simulink model "RVC_Joint_space_PD_control_gravity_compensation"  (R2020b)
settings: Solver=VariableStepAuto  StartTime=0.0  StopTime=10  RelTol=1e-3
values from neighbouring files (symbols this model uses):
  dotqd = [0 0 0 0 0 0]'    [RVC_main.m]
  gravity = [0 0 9.81]'    [RVC_main.m]
  KD_J = diag([1 1 1 0.1 0.1 0.1])    [RVC_main.m]
  KP_J = diag([0.5 0.5 0.5 0.25 0.255 0.25])    [RVC_main.m]
  qd = [0 0 0 0 0 0]'    [RVC_main.m]    (also in forward_dynamics.m = y(:, n+1:2*n)'; forward_recursive_NewtonEulero.m = qd0 + (1.0/6.0)*(M0 + 2*M1 + 2*M2 + M3); inv_dyn_recursive_NewtonEulero.m = Qd')
undefined symbols (not defined in the file or in its folder): dh, inv_dyn_recursive_NewtonEulero
libraries: vrlib x1
settings Model: Creator=eros  LastModifiedBy=nicol

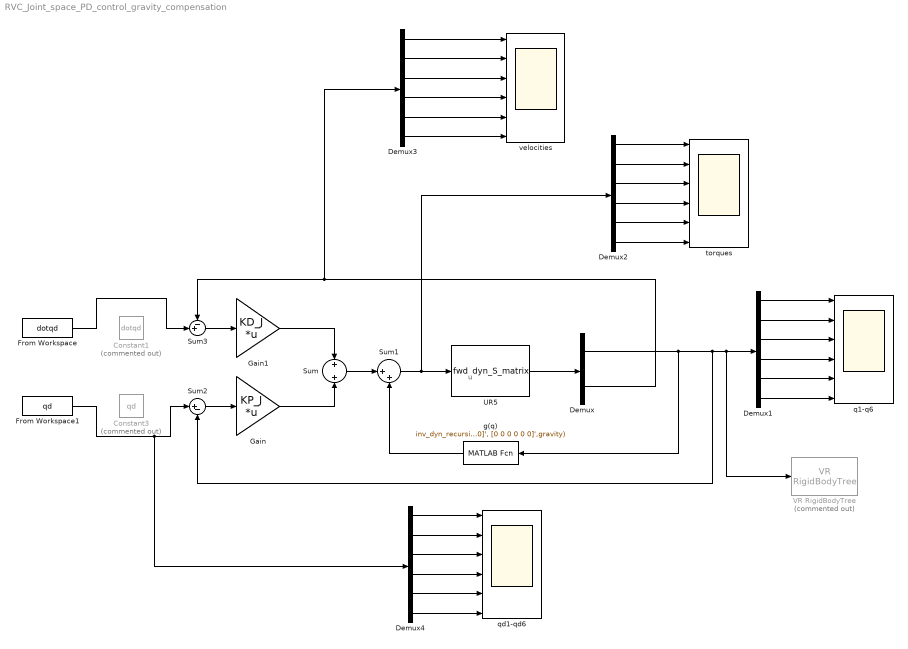
== system RVC_Joint_space_PD_control_gravity_compensation ==
  note: u
  Constant1 : Constant  Commented=on  Value=dotqd
  Constant3 : Constant  Commented=on  Value=qd
  Demux : Demux  Outputs=2
  Demux{1..4} (4 alike) : Demux  Outputs=dh.dof
  From Workspace : FromWorkspace  VariableName=dotqd
  From Workspace1 : FromWorkspace  VariableName=qd
  Gain : Gain  Gain=KP_J  Multiplication=Matrix(K*u)
  Gain1 : Gain  Gain=KD_J  Multiplication=Matrix(K*u)
  Sum : Sum
  Sum1 : Sum  Inputs=|++
  Sum2 : Sum  Inputs=|+-
  Sum3 : Sum  Inputs=-+|
  UR5 : S-Function  FunctionName=fwd_dyn_S_matrix  Parameters=dh, he, gravity, q0, dotq0  SFunctionDeploymentMode=off  EnableBusSupport=off
  VR RigidBodyTree : vrlib/VR RigidBodyTree  Commented=on  RBT=UR5_robot  useRBT=on  Ts=-1  ForceViewerOpen=on
      settings: SourceProductBaseCode=SL
  g(q) : MATLABFcn  MATLABFcn=inv_dyn_recursive_NewtonEulero(dh,u,[0 0 0 0 0 0]', [0 0 0 0 0 0]',gravity)  OutputDimensions=[dh.dof 1]  Output1D=off
  q1-q6 : Scope  NumInputPorts=6
  qd1-qd6 : Scope  NumInputPorts=6
  torques : Scope  NumInputPorts=6
  velocities : Scope  NumInputPorts=6
  wires:
  Sum/1 -> Sum1/1
  g(q)/1 -> Sum1/2
  UR5/1 -> Demux/1
  Demux/1 -> Sum2/2, VR RigidBodyTree/1, Demux1/1, g(q)/1
  Sum2/1 -> Gain/1
  Gain1/1 -> Sum/1
  Demux1/1 -> q1-q6/1
  Demux1/2 -> q1-q6/2
  Demux1/3 -> q1-q6/3
  Demux1/4 -> q1-q6/4
  Demux1/5 -> q1-q6/5
  Demux1/6 -> q1-q6/6
  Sum3/1 -> Gain1/1
  Demux2/6 -> torques/6
  Demux2/5 -> torques/5
  Demux2/3 -> torques/3
  Demux2/4 -> torques/4
  Demux2/1 -> torques/1
  Sum1/1 -> UR5/1, Demux2/1
  Demux2/2 -> torques/2
  Demux3/6 -> velocities/6
  Demux3/5 -> velocities/5
  Demux3/3 -> velocities/3
  Demux3/4 -> velocities/4
  Demux3/1 -> velocities/1
  Demux/2 -> Sum3/1, Demux3/1
  Demux3/2 -> velocities/2
  From Workspace/1 -> Sum3/2
  From Workspace1/1 -> Demux4/1, Sum2/1
  Demux4/4 -> qd1-qd6/4
  Demux4/5 -> qd1-qd6/5
  Demux4/3 -> qd1-qd6/3
  Demux4/2 -> qd1-qd6/2
  Gain/1 -> Sum/2
  Demux4/1 -> qd1-qd6/1
  Demux4/6 -> qd1-qd6/6
